simulink model "PosControl_Quadruped_v3_turn"  (R2018b)
settings: Solver=FixedStepAuto  StartTime=0.0  StopTime=10  FixedStep=0.001  RelTol=1e-3  EnableMultiTasking=on
undefined symbols (not defined in the file or in its folder): X, Y, Z
libraries: sm_lib x43, nesl_utility x39, Contact_Forces_Lib x4, simulink x1
(part 3 of 3)

== matlab function PosControl_Quadruped_v3_turn/controller/trajectory generate3 ==
  data: t input; LegFL output; LegFR output; LegRR output; LegRL output
function [LegFL,LegFR,LegRR,LegRL] = Turn(t)

lamda = 0.5;%摆动周期占比
Ts = 1;%周期时间

Xs = 0;%x轴起点
% XeF = 0.03;
% XeB = -0.05;%

Ys = 0;%y轴起点
% YeL = 0.05;
% YeR = -0.05;%y轴右转终点

H = 0.2;%抬腿高度
Zs = -0.7;%z轴起点

body_len_half = 0.6;
body_width_half = 0.25;
body_diag_half = sqrt(body_len_half*body_width_half);
body_angle_S = atan(body_width_half/body_len_half);
body_angle_L = atan(body_len_half/body_width_half);

O_FL = [body_len_half,body_width_half,Zs,1]';
O_FR = [body_len_half,-body_width_half,Zs,1]';
O_RR = [-body_len_half,-body_width_half,Zs,1]';
O_RL = [-body_len_half,body_width_half,Zs,1]';

FL = [body_len_half,body_width_half,0]';
FR = [body_len_half,-body_width_half,0]';
RR = [-body_len_half,-body_width_half,0]';
RL = [-body_len_half,body_width_half,0]';

FL_trans = [eye(3,3),FL;
    zeros(1,3),1];
FR_trans = [eye(3,3),FR;
    zeros(1,3),1];
RR_trans = [eye(3,3),RR;
    zeros(1,3),1];
RL_trans = [eye(3,3),RL;
    zeros(1,3),1];

if t>0 && t<=lamda*Ts
    time_ratio = t/lamda*Ts;
    yaw = -time_ratio*(5*pi/180);
    
    delta_x = abs(body_diag_half*cos(5*pi/180+body_angle_S)-body_len_half);
    delta_y = abs(body_diag_half*sin(5*pi/180+body_angle_S)-body_width_half);
    
    sigma = 2*pi*t/(lamda*Ts);
    
    x_f = (delta_x-Xs)*((sigma-sin(sigma))/(2*pi))+Xs;  
    y_l = (delta_y-Ys)*((sigma-sin(sigma))/(2*pi))+Ys;

       
    z_up = H*(1-cos(sigma))/2+Zs;
    
    R_yaw = [cos(yaw),-sin(yaw),0,0;
        sin(yaw),cos(yaw),0,0;
        0,0,1,0;
        0,0,0,1];
    
    P_FL_all = inv(FL_trans)*R_yaw*O_FL;
    P_FR_all = inv(FR_trans)*R_yaw*O_FR;
    P_RR_all = inv(RR_trans)*R_yaw*O_RR;
    P_RL_all = inv(RL_trans)*R_yaw*O_RL;

    yawFL = P_FL_all(1:3)';
    yawFR = P_FR_all(1:3)';
    yawRR = P_RR_all(1:3)';
    yawRL = P_RL_all(1:3)';
   
    LegFL = [Xs,Ys,z_up];  
    LegFR = yawFR;
    LegRR = [Xs,Ys,z_up];
    LegRL = yawRL;

    
elseif t>lamda*Ts && t<Ts
    
    time_ratio = (t-lamda*Ts)/(Ts-lamda*Ts);
    yaw = -time_ratio*(5*pi/180);
    
    delta_x = abs(body_diag_half*cos(5*pi/180+body_angle_L)-body_len_half);
    delta_y = abs(body_diag_half*sin(5*pi/180+body_angle_L)-body_width_half);

    sigma = 2*pi*(t-lamda*Ts)/(lamda*Ts);
    x_f = (delta_x-Xs)*((sigma-sin(sigma))/(2*pi))+Xs;  
    y_l = (delta_y-Ys)*((sigma-sin(sigma))/(2*pi))+Ys;
    
    z_up = H*(1-cos(sigma))/2+Zs;
    
    R_yaw = [cos(yaw),-sin(yaw),0,0;
        sin(yaw),cos(yaw),0,0;
        0,0,1,0;
        0,0,0,1];
    
    P_FL_all = inv(FL_trans)*R_yaw*O_FL;
    P_FR_all = inv(FR_trans)*R_yaw*O_FR;
    P_RR_all = inv(RR_trans)*R_yaw*O_RR;
    P_RL_all = inv(RL_trans)*R_yaw*O_RL;

    yawFL = P_FL_all(1:3)';
    yawFR = P_FR_all(1:3)';
    yawRR = P_RR_all(1:3)';
    yawRL = P_RL_all(1:3)';
    
    
    LegFL = yawFL;
    LegFR = [Xs,Ys,z_up];
    LegRR = yawRR;
    LegRL = [Xs,Ys,z_up];
    
else
    LegFL = [Xs,Ys,Zs];  
    LegFR = [Xs,Ys,Zs];
    LegRR = [Xs,Ys,Zs];
    LegRL = [Xs,Ys,Zs];
end

== matlab function PosControl_Quadruped_v3_turn/controller/trajectory generate1 ==
  data: roll input; pitch input; yaw input; t input; LegFL output; LegFR output; LegRR output; LegRL output
function [LegFL,LegFR,LegRR,LegRL] = gesture(roll,pitch,yaw,t)

Xs = 0;
Ys = 0;
Zs = -0.7;

if t>2
    O_FL = [0.6,0.25,-0.7,1]';
    O_FR = [0.6,-0.25,-0.7,1]';
    O_RR = [-0.6,-0.25,-0.7,1]';
    O_RL = [-0.6,0.25,-0.7,1]';
    
    FL = [0.6,0.25,0]';
    FR = [0.6,-0.25,0]';
    RR = [-0.6,-0.25,0]';
    RL = [-0.6,0.25,0]';
    
    FL_trans = [eye(3,3),FL;
        zeros(1,3),1];
    FR_trans = [eye(3,3),FR;
        zeros(1,3),1];
    RR_trans = [eye(3,3),RR;
        zeros(1,3),1];
    RL_trans = [eye(3,3),RL;
        zeros(1,3),1];
    
    R_roll = [ 1,0,0,0;
        0,cos(roll),-sin(roll),0;
        0,sin(roll),cos(roll),0;
        0,0,0,1];
    
    R_pitch = [cos(pitch),0,sin(pitch),0;
        0,1,0,0;
        -sin(pitch),0,cos(pitch),0;
        0,0,0,1];
    
    R_yaw = [cos(yaw),-sin(yaw),0,0;
        sin(yaw),cos(yaw),0,0;
        0,0,1,0;
        0,0,0,1];
    
    
%     P_FL_roll = inv(FL_trans)*R_roll*O_FL;
%     P_FL_pitch = inv(FL_trans)*R_pitch*O_FL;
%     P_FL_yaw = inv(FL_trans)*R_yaw*O_FL;
%     
%     P_FR_roll = inv(FR_trans)*R_roll*O_FR;
%     P_FR_pitch = inv(FR_trans)*R_pitch*O_FR;
%     P_FR_yaw = inv(FR_trans)*R_yaw*O_FR;
%     
%     P_RR_roll = inv(RR_trans)*R_roll*O_RR;
%     P_RR_pitch = inv(RR_trans)*R_pitch*O_RR;
%     P_RR_yaw = inv(RR_trans)*R_yaw*O_RR;
%     
%     P_RL_roll = inv(RL_trans)*R_roll*O_RL;
%     P_RL_pitch = inv(RL_trans)*R_pitch*O_RL;
%     P_RL_yaw = inv(RL_trans)*R_yaw*O_RL;
    
    P_FL_all = inv(FL_trans)*R_roll*R_pitch*R_yaw*O_FL;
    P_FR_all = inv(FR_trans)*R_roll*R_pitch*R_yaw*O_FR;
    P_RR_all = inv(RR_trans)*R_roll*R_pitch*R_yaw*O_RR;
    P_RL_all = inv(RL_trans)*R_roll*R_pitch*R_yaw*O_RL;
    
    
%     LegFL = P_FL_roll(1:3)';
%     LegFR = P_FR_roll(1:3)';
%     LegRR = P_RR_roll(1:3)';
%     LegRL = P_RL_roll(1:3)';
    
%     LegFL = P_FL_pitch(1:3)';
%     LegFR = P_FR_pitch(1:3)';
%     LegRR = P_RR_pitch(1:3)';
%     LegRL = P_RL_pitch(1:3)';

%     LegFL = P_FL_yaw(1:3)';
%     LegFR = P_FR_yaw(1:3)';
%     LegRR = P_RR_yaw(1:3)';
%     LegRL = P_RL_yaw(1:3)';

    LegFL = P_FL_all(1:3)';
    LegFR = P_FR_all(1:3)';
    LegRR = P_RR_all(1:3)';
    LegRL = P_RL_all(1:3)';
else
    LegFL = [Xs,Ys,Zs];
    LegFR = [Xs,Ys,Zs];
    LegRR = [Xs,Ys,Zs];
    LegRL = [Xs,Ys,Zs];
end

== matlab function PosControl_Quadruped_v3_turn/controller/inverse kinematics2 ==
  data: x input; y input; z input; shoulder output; hip output; knee output
function [shoulder,hip,knee]= coord2theta(x,y,z)
% L1=75.0;
% L2=415.0;
% L3=408.0;


% temp = (L1*L1+L2*L2-x*x-z*z)/(2*L1*L2);
% if temp>1
%     temp = 1;
% elseif temp<-1
%     temp=1;
% end
% theta2 = pi-acos(temp);
% 
% temp = (x*x+z*z+L1*L1-L2*L2)/(2*sqrt(x*x+z*z)*L1);
% if temp>1
%     temp = 1;
% elseif temp<-1
%     temp=1;
% end
% if(x>0)
%     theta1 = abs(atan(x/z))-acos(temp);
% elseif(x<0)
%     theta1 = -abs(atan(x/z))-acos(temp);
% else
%     theta1 = -acos(temp);

L1=0;
L2=0.5;
L3=0.5;

shoulder=atan(-y/z);

%髋关节到足端长度的平方
L_H2E_2=x*x+(y-L1*sin(shoulder))*(y-L1*sin(shoulder))+(z+L1*cos(shoulder))*(z+L1*cos(shoulder));
%髋关节到足端长度
L_H2E=sqrt(L_H2E_2);

temp = (L2*L2+L_H2E_2-L3*L3)/(2*L_H2E*L2);
if temp>1
    temp = 1;
elseif temp<-1
    temp = -1;
end
Zeta=acos(temp);
hip=atan(x/(sqrt(y*y+z*z)-L1))-Zeta;

temp = (L2*L2+L3*L3-L_H2E_2)/(2*L2*L3);
if temp>1
    temp = 1;
elseif temp<-1
    temp = -1;
end
knee=pi-acos(temp);

== matlab function PosControl_Quadruped_v3_turn/controller/inverse kinematics3 ==
  data: x input; y input; z input; shoulder output; hip output; knee output
function [shoulder,hip,knee]= coord2theta(x,y,z)
% L1=75.0;
% L2=415.0;
% L3=408.0;


% temp = (L1*L1+L2*L2-x*x-z*z)/(2*L1*L2);
% if temp>1
%     temp = 1;
% elseif temp<-1
%     temp=1;
% end
% theta2 = pi-acos(temp);
% 
% temp = (x*x+z*z+L1*L1-L2*L2)/(2*sqrt(x*x+z*z)*L1);
% if temp>1
%     temp = 1;
% elseif temp<-1
%     temp=1;
% end
% if(x>0)
%     theta1 = abs(atan(x/z))-acos(temp);
% elseif(x<0)
%     theta1 = -abs(atan(x/z))-acos(temp);
% else
%     theta1 = -acos(temp);

L1=0;
L2=0.5;
L3=0.5;

shoulder=atan(-y/z);

%髋关节到足端长度的平方
L_H2E_2=x*x+(y-L1*sin(shoulder))*(y-L1*sin(shoulder))+(z+L1*cos(shoulder))*(z+L1*cos(shoulder));
%髋关节到足端长度
L_H2E=sqrt(L_H2E_2);

temp = (L2*L2+L_H2E_2-L3*L3)/(2*L_H2E*L2);
if temp>1
    temp = 1;
elseif temp<-1
    temp = -1;
end
Zeta=acos(temp);
hip=atan(x/(sqrt(y*y+z*z)-L1))-Zeta;

temp = (L2*L2+L3*L3-L_H2E_2)/(2*L2*L3);
if temp>1
    temp = 1;
elseif temp<-1
    temp = -1;
end
knee=pi-acos(temp);

== matlab function PosControl_Quadruped_v3_turn/controller/inverse kinematics4 ==
  data: x input; y input; z input; shoulder output; hip output; knee output
function [shoulder,hip,knee]= coord2theta(x,y,z)
% L1=75.0;
% L2=415.0;
% L3=408.0;


% temp = (L1*L1+L2*L2-x*x-z*z)/(2*L1*L2);
% if temp>1
%     temp = 1;
% elseif temp<-1
%     temp=1;
% end
% theta2 = pi-acos(temp);
% 
% temp = (x*x+z*z+L1*L1-L2*L2)/(2*sqrt(x*x+z*z)*L1);
% if temp>1
%     temp = 1;
% elseif temp<-1
%     temp=1;
% end
% if(x>0)
%     theta1 = abs(atan(x/z))-acos(temp);
% elseif(x<0)
%     theta1 = -abs(atan(x/z))-acos(temp);
% else
%     theta1 = -acos(temp);

L1=0;
L2=0.5;
L3=0.5;

shoulder=atan(-y/z);

%髋关节到足端长度的平方
L_H2E_2=x*x+(y-L1*sin(shoulder))*(y-L1*sin(shoulder))+(z+L1*cos(shoulder))*(z+L1*cos(shoulder));
%髋关节到足端长度
L_H2E=sqrt(L_H2E_2);

temp = (L2*L2+L_H2E_2-L3*L3)/(2*L_H2E*L2);
if temp>1
    temp = 1;
elseif temp<-1
    temp = -1;
end
Zeta=acos(temp);
hip=atan(x/(sqrt(y*y+z*z)-L1))-Zeta;

temp = (L2*L2+L3*L3-L_H2E_2)/(2*L2*L3);
if temp>1
    temp = 1;
elseif temp<-1
    temp = -1;
end
knee=pi-acos(temp);

== matlab function PosControl_Quadruped_v3_turn/controller/inverse kinematics5 ==
  data: x input; y input; z input; shoulder output; hip output; knee output
function [shoulder,hip,knee]= coord2theta(x,y,z)
% L1=75.0;
% L2=415.0;
% L3=408.0;


% temp = (L1*L1+L2*L2-x*x-z*z)/(2*L1*L2);
% if temp>1
%     temp = 1;
% elseif temp<-1
%     temp=1;
% end
% theta2 = pi-acos(temp);
% 
% temp = (x*x+z*z+L1*L1-L2*L2)/(2*sqrt(x*x+z*z)*L1);
% if temp>1
%     temp = 1;
% elseif temp<-1
%     temp=1;
% end
% if(x>0)
%     theta1 = abs(atan(x/z))-acos(temp);
% elseif(x<0)
%     theta1 = -abs(atan(x/z))-acos(temp);
% else
%     theta1 = -acos(temp);

L1=0;
L2=0.5;
L3=0.5;

shoulder=atan(-y/z);

%髋关节到足端长度的平方
L_H2E_2=x*x+(y-L1*sin(shoulder))*(y-L1*sin(shoulder))+(z+L1*cos(shoulder))*(z+L1*cos(shoulder));
%髋关节到足端长度
L_H2E=sqrt(L_H2E_2);

temp = (L2*L2+L_H2E_2-L3*L3)/(2*L_H2E*L2);
if temp>1
    temp = 1;
elseif temp<-1
    temp = -1;
end
Zeta=acos(temp);
hip=atan(x/(sqrt(y*y+z*z)-L1))-Zeta;

temp = (L2*L2+L3*L3-L_H2E_2)/(2*L2*L3);
if temp>1
    temp = 1;
elseif temp<-1
    temp = -1;
end
knee=pi-acos(temp);

== matlab function PosControl_Quadruped_v3_turn/controller/trajectory generate2 ==
  data: timer1 output; timer2 output; timer1 input; LegFL output; LegFR output; LegRR output; LegRL output; timer2 input
function [timer1,timer2,LegFL,LegFR,LegRR,LegRL] = Turn(timer1,timer2)

lamda = 0.5;%摆动周期占比
Ts = 1;%周期时间

if timer2<1.5
    timer2 = timer2+0.001;
else
    timer1=timer1+0.001;
    if timer1>=Ts
        timer1=0;
    end
end

Xs = -0.15;%x轴起点
XeF = 0.1;
XeB = -0.2;
% XeF = 0.03;
% XeB = -0.05;

Ys = 0;%y轴起点
% YeL = 0.05;
% YeR = -0.05;

H = 0.2;%抬腿高度
Zs = -0.7;%z轴起点

body_len_half = 0.6;
body_width_half = 0.25;
body_diag_half = sqrt(body_len_half*body_width_half);
body_angle_S = atan(body_width_half/body_len_half);
body_angle_L = atan(body_len_half/body_width_half);

% O_FL = [body_len_half,body_width_half,Zs,1]';
% O_FR = [body_len_half,-body_width_half,Zs,1]';
% O_RR = [-body_len_half,-body_width_half,Zs,1]';
% O_RL = [-body_len_half,body_width_half,Zs,1]';
% 
% FL = [body_len_half,body_width_half,0]';
% FR = [body_len_half,-body_width_half,0]';
% RR = [-body_len_half,-body_width_half,0]';
% RL = [-body_len_half,body_width_half,0]';
% 
% FL_trans = [eye(3,3),FL;
%     zeros(1,3),1];
% FR_trans = [eye(3,3),FR;
%     zeros(1,3),1];
% RR_trans = [eye(3,3),RR;
%     zeros(1,3),1];
% RL_trans = [eye(3,3),RL;
%     zeros(1,3),1];

if timer1 == 0 && timer2 >=1
    
    sigma = 2*pi*(timer2-1)/(lamda*Ts);
    x_f = (XeF-Xs)*((sigma-sin(sigma))/(2*pi))+Xs;  
    z_up = H*(1-cos(sigma))/2+Zs;
    LegFL = [Xs,Ys,Zs];  
    LegFR = [x_f,Ys,z_up];
    LegRR = [Xs,Ys,Zs];
    LegRL = [x_f,Ys,z_up];

    
elseif timer1>0 && timer1<=lamda*Ts
%     time_ratio = t/lamda*Ts;
%     yaw = -time_ratio*(5*pi/180);
    
    delta_x = abs(body_diag_half*cos(5*pi/180+body_angle_S)-body_len_half);
    delta_y = abs(body_diag_half*sin(5*pi/180+body_angle_S)-body_width_half);
    
    sigma = 2*pi*timer1/(lamda*Ts);
    
%     x_f = (delta_x-Xs)*((sigma-sin(sigma))/(2*pi))+Xs;  
%     y_l = (delta_y-Ys)*((sigma-sin(sigma))/(2*pi))+Ys;

    x_f = (XeF-Xs)*((sigma-sin(sigma))/(2*pi))+Xs;  
    x_fb = (Xs-XeF)*((sigma-sin(sigma))/(2*pi))+XeF;  
%     
%     x_b = (XeB-Xs)*((sigma-sin(sigma))/(2*pi))+Xs;  
%     x_bb = (Xs-XeB)*((sigma-sin(sigma))/(2*pi))+XeB;
    
    z_up = H*(1-cos(sigma))/2+Zs;
    
%     R_yaw = [cos(yaw),-sin(yaw),0,0;
%         sin(yaw),cos(yaw),0,0;
%         0,0,1,0;
%         0,0,0,1];
%     
%     P_FL_all = inv(FL_trans)*R_yaw*O_FL;
%     P_FR_all = inv(FR_trans)*R_yaw*O_FR;
%     P_RR_all = inv(RR_trans)*R_yaw*O_RR;
%     P_RL_all = inv(RL_trans)*R_yaw*O_RL;
% 
%     yawFL = P_FL_all(1:3)';
%     yawFR = P_FR_all(1:3)';
%     yawRR = P_RR_all(1:3)';
%     yawRL = P_RL_all(1:3)';
   
%     LegFL = [-x_f,y_l,z_up];  
%     LegFR = [Xs,Ys,Zs];
%     LegRR = [x_f,-y_l,z_up];
%     LegRL = [Xs,Ys,Zs];
    
    LegFL = [x_f,Ys,z_up];  
    LegFR = [x_fb,Ys,Zs];
    LegRR = [x_f,Ys,z_up];
    LegRL = [x_fb,Ys,Zs];
    
elseif timer1>lamda*Ts && timer1<Ts
    
%     time_ratio = (t-lamda*Ts)/(Ts-lamda*Ts);
%     yaw = -time_ratio*(5*pi/180);
    
    delta_x = abs(body_diag_half*cos(5*pi/180+body_angle_S)-body_len_half);
    delta_y = abs(body_diag_half*sin(5*pi/180+body_angle_S)-body_width_half);

    sigma = 2*pi*(timer1-lamda*Ts)/(lamda*Ts);
%     x_f = (delta_x-Xs)*((sigma-sin(sigma))/(2*pi))+Xs;  
%     y_l = (delta_y-Ys)*((sigma-sin(sigma))/(2*pi))+Ys;
    
    x_f = (XeF-Xs)*((sigma-sin(sigma))/(2*pi))+Xs;  
    x_fb = (Xs-XeF)*((sigma-sin(sigma))/(2*pi))+XeF;  
    
%     x_b = (XeB-Xs)*((sigma-sin(sigma))/(2*pi))+Xs;  
%     x_bb = (Xs-XeB)*((sigma-sin(sigma))/(2*pi))+XeB;
    
    z_up = H*(1-cos(sigma))/2+Zs;
    
%     R_yaw = [cos(yaw),-sin(yaw),0,0;
%         sin(yaw),cos(yaw),0,0;
%         0,0,1,0;
%         0,0,0,1];
%     
%     P_FL_all = inv(FL_trans)*R_yaw*O_FL;
%     P_FR_all = inv(FR_trans)*R_yaw*O_FR;
%     P_RR_all = inv(RR_trans)*R_yaw*O_RR;
%     P_RL_all = inv(RL_trans)*R_yaw*O_RL;
% 
%     yawFL = P_FL_all(1:3)';
%     yawFR = P_FR_all(1:3)';
%     yawRR = P_RR_all(1:3)';
%     yawRL = P_RL_all(1:3)';
    
    LegFL = [x_fb,Ys,Zs];
    LegFR = [x_f,Ys,z_up];
    LegRR = [x_fb,Ys,Zs];
    LegRL = [x_f,Ys,z_up];
    
else
    LegFL = [Xs,Ys,Zs];  
    LegFR = [Xs,Ys,Zs];
    LegRR = [Xs,Ys,Zs];
    LegRL = [Xs,Ys,Zs];
end
